simulink model "Simulation"  (R2016a)
settings: Solver=FixedStepAuto  StartTime=0.0  StopTime=20  FixedStep=0.01  RelTol=1e-3
undefined symbols (not defined in the file or in its folder): beta, g0, g1, g2, g3, gamma, kappa, landa, nu
(part 28 of 30)

== matlab function Simulation/e edot to sp ==
  data: despar input; e input; edot input; z1 output; z2 output; z3 output; z4 output; z5 output; z6 output
function [z1 ,z2, z3, z4, z5 ,z6]    = fcn(despar,e,edot)

z1=despar(1)*((abs(e(1)))^despar(5))*sign(e(1))+despar(2)*e(1)+...
    despar(3)*(e(1)^3)+despar(4)*despar(6)*(abs(e(1)))^(despar(6)-1)*edot(1);

z2=despar(1)*((abs(e(2)))^despar(5))*sign(e(2))+despar(2)*e(2)+...
    despar(3)*(e(2)^3)+despar(4)*despar(6)*(abs(e(2)))^(despar(6)-1)*edot(2);

z3=despar(1)*((abs(e(3)))^despar(5))*sign(e(3))+despar(2)*e(3)+...
    despar(3)*(e(3)^3)+despar(4)*despar(6)*(abs(e(3)))^(despar(6)-1)*edot(3);

z4=despar(1)*((abs(e(4)))^despar(5))*sign(e(4))+despar(2)*e(4)+...
    despar(3)*(e(4)^3)+despar(4)*despar(6)*(abs(e(4)))^(despar(6)-1)*edot(4);

z5=despar(1)*((abs(e(5)))^despar(5))*sign(e(5))+despar(2)*e(5)+...
    despar(3)*(e(5)^3)+despar(4)*despar(6)*(abs(e(5)))^(despar(6)-1)*edot(5);

z6=despar(1)*((abs(e(6)))^despar(5))*sign(e(6))+despar(2)*e(6)+...
    despar(3)*(e(6)^3)+despar(4)*despar(6)*(abs(e(6)))^(despar(6)-1)*edot(6);
